simulink model "A_Justo_SCHFV_slx_IV"  (R2019a)
settings: Solver=VariableStepAuto  StartTime=0.0  StopTime=tfinal  MaxStep=maxstepsize  RelTol=1e-3  EnableMultiTasking=on
values from neighbouring files (symbols this model uses):
  aini = 0    [A_Justo_SCHFV_m_UFHDV_Design.m]
  B = [0; 0; 0; 0; 1/Tau_A]    [A_Justo_SCHFV_m_Control_Sensitivity.m]    (also in A_Justo_SCHFV_m_UFHDV_Design.m; TransferFunctionPROP.m)
  IDM_Amax = IDM_Amax(acc1+n1,acc1+n1)    [TransferFunctionPROP.m]
  IDM_Delta = IDM_Delta(acc1+n1)    [TransferFunctionPROP.m]
  IDM_H0 = IDM_H0(acc1+n1)    [TransferFunctionPROP.m]
  IDM_T = normrnd(IDM_t,IDM_ts)    [A_Justo_SCHFV_m_Control_Sensitivity.m]    (also in A_Justo_SCHFV_m_Track.m = IDM_Tind; A_Justo_SCHFV_m_UFHDV_Design.m; TransferFunctionPROP.m = IDM_T(acc1+n1,acc1+n1))
  IDM_V0 = IDM_V0(acc1+n1)    [TransferFunctionPROP.m]
  L = Lini    [A_Justo_SCHFV_m_Track.m]
  N = 11    [A_Justo_SCHFV_m_IV.m]    (also in A_Justo_SCHFV_m_Track.m)
  R = d/(2*pi)    (= 31.8309886184)    [A_Justo_SCHFV_m_IV.m]    (also in A_Justo_SCHFV_m_Track.m)
  Sidm = diag(isIDM)    [A_Justo_SCHFV_m_IV.m]    (also in A_Justo_SCHFV_m_Track.m)
  Smit = diag(isMIT)    [A_Justo_SCHFV_m_IV.m]    (also in A_Justo_SCHFV_m_Track.m)
  vini = 0    [A_Justo_SCHFV_m_UFHDV_Design.m]
undefined symbols (not defined in the file or in its folder): Bv, IDM_iSqab, iTau, MITSIM_a_Free_bra_high, MITSIM_a_Free_bra_low, MITSIM_a_Free_bra_mid, MITSIM_a_Free_bra_midhigh, MITSIM_a_Free_bra_midlow, MITSIM_a_Free_thr_high, MITSIM_a_Free_thr_low, MITSIM_a_Free_thr_mid, MITSIM_Alpha_bra, MITSIM_Alpha_thr, MITSIM_Beta_bra, MITSIM_Beta_thr, MITSIM_Gamma_bra, MITSIM_Gamma_thr, MITSIM_T_lower, MITSIM_T_upper, thini
settings Model: Creator=arnaudoria  LastModifiedBy=Sander
settings DataIOCC: LimitDataPoints=on  ReturnWorkspaceOutputs=off
settings OptimizationCC: LifeSpan=inf
settings DebuggingCC: AllowSymbolicDim=off  SFUnexpectedBacktrackingDiag=warning  SFNoUnconditionalDefaultTransitionDiag=warning  SFExecutionAtInitializationDiag=none  ArithmeticOperatorsInVariantConditions=warning
settings ModelReferenceCC: PropagateSignalLabelsOutOfModel=off
settings SFSimCC: SimUseLocalCustomCode=off
settings RTWCC: RTWUseLocalCustomCode=off
settings CodeAppCC: StateflowObjectComments=on
settings GRTTargetCC: TargetLangStandard=C89/C90 (ANSI)
settings ConfigComp: CovMetricSettings=dw  CovHtmlReporting=on  CovSaveCumulativeToWorkspaceVar=on  CovSaveSingleToWorkspaceVar=on  CovExternalEMLEnable=off

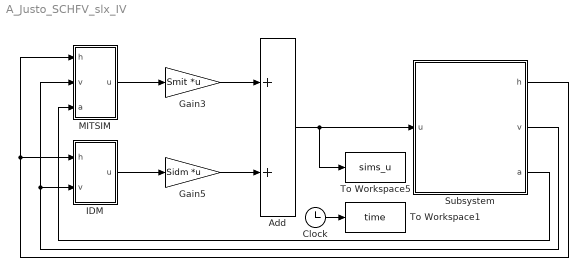
== system A_Justo_SCHFV_slx_IV ==
  Add : Sum
  Clock : Clock
  Gain3 : Gain  Gain=Smit  Multiplication=Matrix(K*u)
  Gain5 : Gain  Gain=Sidm  Multiplication=Matrix(K*u)
  IDM : Subsystem
  MITSIM : Subsystem
  Subsystem : Subsystem
  To Workspace1 : ToWorkspace  VariableName=time  SampleTime=-1
  To Workspace5 : ToWorkspace  VariableName=sims_u  SampleTime=-1
  wires:
  Clock/1 -> To Workspace1/1
  Subsystem/1(h) -> MITSIM/1(h), IDM/1(h)
  Subsystem/2(v) -> IDM/2(v), MITSIM/2(v)
  Subsystem/3(a) -> MITSIM/3(a)
  Add/1 -> Subsystem/1(u), To Workspace5/1
  Gain5/1 -> Add/2
  IDM/1(u) -> Gain5/1
  MITSIM/1(u) -> Gain3/1
  Gain3/1 -> Add/1

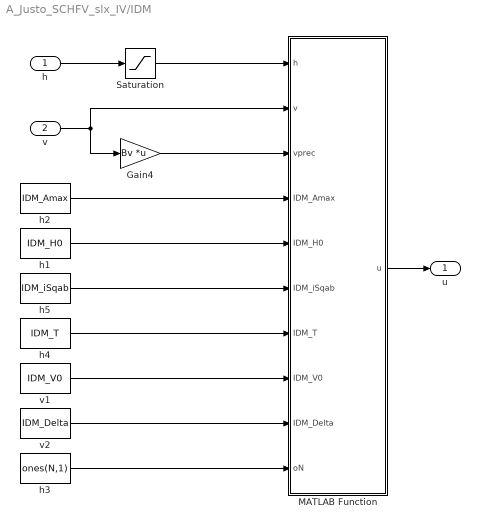
== system A_Justo_SCHFV_slx_IV/IDM ==
  h : Inport
  v : Inport  Port=2
  Gain4 : Gain  Gain=Bv  Multiplication=Matrix(K*u)
  MATLAB Function : MATLAB Function  TreatAsAtomicUnit=on
  Saturation : Saturate  UpperLimit=inf  LowerLimit=0.1
  h1 : Constant  Value=IDM_H0
  h2 : Constant  Value=IDM_Amax
  h3 : Constant  Value=ones(N,1)
  h4 : Constant  Value=IDM_T
  h5 : Constant  Value=IDM_iSqab
  v1 : Constant  Value=IDM_V0
  v2 : Constant  Value=IDM_Delta
  u : Outport
  wires:
  v/1 -> Gain4/1, MATLAB Function/2(v)
  v2/1 -> MATLAB Function/9(IDM_Delta)
  Gain4/1 -> MATLAB Function/3(vprec)
  h5/1 -> MATLAB Function/6(IDM_iSqab)
  MATLAB Function/1(u) -> u/1
  h4/1 -> MATLAB Function/7(IDM_T)
  h3/1 -> MATLAB Function/10(oN)
  Saturation/1 -> MATLAB Function/1(h)
  h/1 -> Saturation/1
  h1/1 -> MATLAB Function/5(IDM_H0)
  v1/1 -> MATLAB Function/8(IDM_V0)
  h2/1 -> MATLAB Function/4(IDM_Amax)

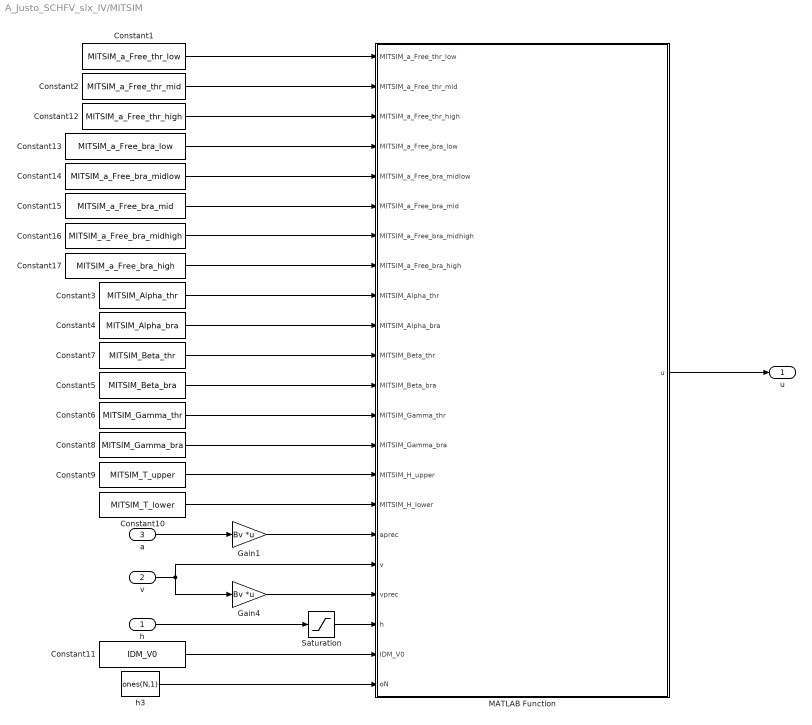
== system A_Justo_SCHFV_slx_IV/MITSIM ==
  h : Inport
  v : Inport  Port=2
  a : Inport  Port=3
  Constant1 : Constant  Value=MITSIM_a_Free_thr_low
  Constant10 : Constant  Value=MITSIM_T_lower
  Constant11 : Constant  Value=IDM_V0
  Constant12 : Constant  Value=MITSIM_a_Free_thr_high
  Constant13 : Constant  Value=MITSIM_a_Free_bra_low
  Constant14 : Constant  Value=MITSIM_a_Free_bra_midlow
  Constant15 : Constant  Value=MITSIM_a_Free_bra_mid
  Constant16 : Constant  Value=MITSIM_a_Free_bra_midhigh
  Constant17 : Constant  Value=MITSIM_a_Free_bra_high
  Constant2 : Constant  Value=MITSIM_a_Free_thr_mid
  Constant3 : Constant  Value=MITSIM_Alpha_thr
  Constant4 : Constant  Value=MITSIM_Alpha_bra
  Constant5 : Constant  Value=MITSIM_Beta_bra
  Constant6 : Constant  Value=MITSIM_Gamma_thr
  Constant7 : Constant  Value=MITSIM_Beta_thr
  Constant8 : Constant  Value=MITSIM_Gamma_bra
  Constant9 : Constant  Value=MITSIM_T_upper
  Gain1 : Gain  Gain=Bv  Multiplication=Matrix(K*u)
  Gain4 : Gain  Gain=Bv  Multiplication=Matrix(K*u)
  MATLAB Function : MATLAB Function  TreatAsAtomicUnit=on
  Saturation : Saturate  UpperLimit=inf  LowerLimit=0.1
  h3 : Constant  Value=ones(N,1)
  u : Outport
  wires:
  Saturation/1 -> MATLAB Function/20(h)
  h/1 -> Saturation/1
  MATLAB Function/1(u) -> u/1
  Gain4/1 -> MATLAB Function/19(vprec)
  v/1 -> Gain4/1, MATLAB Function/18(v)
  Constant1/1 -> MATLAB Function/1(MITSIM_a_Free_thr_low)
  Constant2/1 -> MATLAB Function/2(MITSIM_a_Free_thr_mid)
  Constant3/1 -> MATLAB Function/9(MITSIM_Alpha_thr)
  h3/1 -> MATLAB Function/22(oN)
  a/1 -> Gain1/1
  Gain1/1 -> MATLAB Function/17(aprec)
  Constant4/1 -> MATLAB Function/10(MITSIM_Alpha_bra)
  Constant7/1 -> MATLAB Function/11(MITSIM_Beta_thr)
  Constant5/1 -> MATLAB Function/12(MITSIM_Beta_bra)
  Constant6/1 -> MATLAB Function/13(MITSIM_Gamma_thr)
  Constant8/1 -> MATLAB Function/14(MITSIM_Gamma_bra)
  Constant9/1 -> MATLAB Function/15(MITSIM_H_upper)
  Constant10/1 -> MATLAB Function/16(MITSIM_H_lower)
  Constant11/1 -> MATLAB Function/21(IDM_V0)
  Constant12/1 -> MATLAB Function/3(MITSIM_a_Free_thr_high)
  Constant13/1 -> MATLAB Function/4(MITSIM_a_Free_bra_low)
  Constant14/1 -> MATLAB Function/5(MITSIM_a_Free_bra_midlow)
  Constant15/1 -> MATLAB Function/6(MITSIM_a_Free_bra_mid)
  Constant16/1 -> MATLAB Function/7(MITSIM_a_Free_bra_midhigh)
  Constant17/1 -> MATLAB Function/8(MITSIM_a_Free_bra_high)

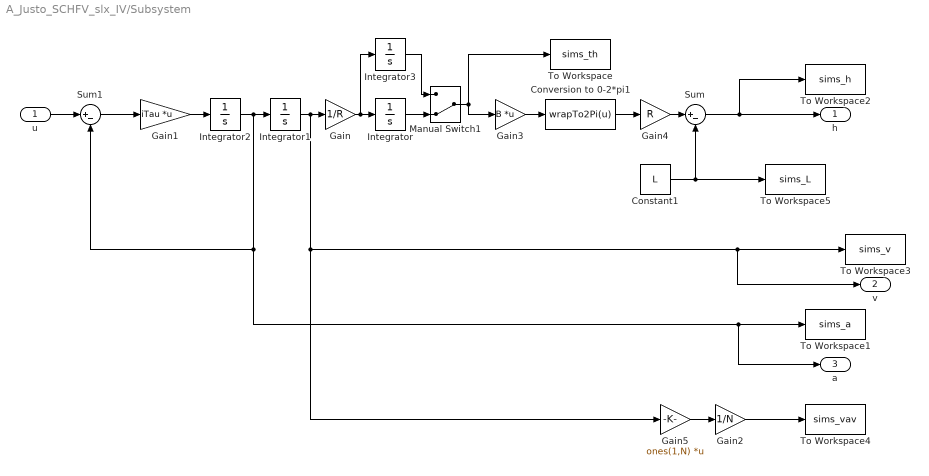
== system A_Justo_SCHFV_slx_IV/Subsystem ==
  u : Inport
  Constant1 : Constant  Value=L
  Conversion to 0-2*pi1 : MATLABFcn  MATLABFcn=wrapTo2Pi(u)
  Gain : Gain  Gain=1/R
  Gain1 : Gain  Gain=iTau  Multiplication=Matrix(K*u)
  Gain2 : Gain  Gain=1/N
  Gain3 : Gain  Gain=B  Multiplication=Matrix(K*u)
  Gain4 : Gain  Gain=R
  Gain5 : Gain  Gain=ones(1,N)  Multiplication=Matrix(K*u)
  Integrator : Integrator  InitialCondition=thini  WrapState=on  WrappedStateUpperValue=2*pi  WrappedStateLowerValue=0
  Integrator1 : Integrator  InitialCondition=vini  LimitOutput=on  LowerSaturationLimit=0  WrappedStateUpperValue=2*pi  WrappedStateLowerValue=0
  Integrator2 : Integrator  InitialCondition=aini  WrappedStateUpperValue=2*pi  WrappedStateLowerValue=0
  Integrator3 : Integrator  InitialCondition=thini  WrappedStateUpperValue=2*pi  WrappedStateLowerValue=0
  Manual Switch1 : ManualSwitch  CurrentSetting=0
  Sum : Sum  Inputs=|+-
  Sum1 : Sum  Inputs=|+-
  To Workspace : ToWorkspace  VariableName=sims_th  SampleTime=-1
  To Workspace1 : ToWorkspace  VariableName=sims_a  SampleTime=-1
  To Workspace2 : ToWorkspace  VariableName=sims_h  SampleTime=-1
  To Workspace3 : ToWorkspace  VariableName=sims_v  SampleTime=-1
  To Workspace4 : ToWorkspace  VariableName=sims_vav  SampleTime=-1
  To Workspace5 : ToWorkspace  VariableName=sims_L  SampleTime=-1
  h : Outport
  v : Outport  Port=2
  a : Outport  Port=3
  wires:
  Gain/1 -> Integrator3/1, Integrator/1
  Gain3/1 -> Conversion to 0-2*pi1/1
  Gain4/1 -> Sum/1
  Sum/1 -> To Workspace2/1, h/1
  u/1 -> Sum1/1
  Integrator1/1 -> Gain5/1, v/1, To Workspace3/1, Gain/1
  Integrator2/1 -> To Workspace1/1, a/1, Sum1/2, Integrator1/1
  Gain1/1 -> Integrator2/1
  Sum1/1 -> Gain1/1
  Integrator3/1 -> Manual Switch1/1
  Integrator/1 -> Manual Switch1/2
  Manual Switch1/1 -> To Workspace/1, Gain3/1
  Conversion to 0-2*pi1/1 -> Gain4/1
  Gain5/1 -> Gain2/1
  Gain2/1 -> To Workspace4/1
  Constant1/1 -> To Workspace5/1, Sum/2

== matlab function A_Justo_SCHFV_slx_IV/IDM/MATLAB Function ==
  data: h input; v input; vprec input; IDM_Amax input; IDM_H0 input; IDM_iSqab input; IDM_T input; IDM_V0 input; IDM_Delta input; u output; oN input
function u = fcn(h,v,vprec,IDM_Amax,IDM_H0,IDM_iSqab,IDM_T,IDM_V0,IDM_Delta,oN)

% IDM
hr = IDM_H0+max(oN*0,IDM_T*v+v.*(v-vprec).*IDM_iSqab);
% Condition for avoiding numerical errors
v = v.*(v>0);
% Control
u = IDM_Amax*(oN-(v./IDM_V0).^IDM_Delta-(hr./h).^2);

== matlab function A_Justo_SCHFV_slx_IV/MITSIM/MATLAB Function ==
  data: MITSIM_a_Free_thr_low input; MITSIM_a_Free_thr_mid input; MITSIM_a_Free_thr_high input; MITSIM_a_Free_bra_low input; MITSIM_a_Free_bra_midlow input; MITSIM_a_Free_bra_mid input; MITSIM_a_Free_bra_midhigh input; MITSIM_a_Free_bra_high input; MITSIM_Alpha_thr input; MITSIM_Alpha_bra input; MITSIM_Beta_thr input; MITSIM_Beta_bra input; MITSIM_Gamma_thr input; MITSIM_Gamma_bra input; MITSIM_H_upper input; MITSIM_H_lower input; aprec input; v input; vprec input; h input; IDM_V0 input; u output; oN input
function u = fcn(MITSIM_a_Free_thr_low, MITSIM_a_Free_thr_mid, ...
    MITSIM_a_Free_thr_high, MITSIM_a_Free_bra_low, ...
    MITSIM_a_Free_bra_midlow, MITSIM_a_Free_bra_mid, ...
    MITSIM_a_Free_bra_midhigh, MITSIM_a_Free_bra_high, MITSIM_Alpha_thr...
    , MITSIM_Alpha_bra, MITSIM_Beta_thr, MITSIM_Beta_bra, ...
MITSIM_Gamma_thr, MITSIM_Gamma_bra, MITSIM_H_upper, MITSIM_H_lower, ...
aprec, v, vprec, h, IDM_V0, oN)

if isempty(find(h<=0, 1))==0  % Display a message to show when some h is not positive
    error('Vehicles have crashed. Simulation has been stopped.')
end

hd_tm = h./v;

% Obtain the indexes that correspond to each regime
ind_free_thr_low = hd_tm>MITSIM_H_upper & v<IDM_V0 & v>12.192;
ind_free_thr_mid = hd_tm>MITSIM_H_upper & v<IDM_V0 & v<=12.192 & v>=6.096;
ind_free_thr_high = hd_tm>MITSIM_H_upper & v<IDM_V0 & v<6.096;
ind_free_zro = hd_tm>MITSIM_H_upper & v==IDM_V0;
ind_free_bra_low = hd_tm>MITSIM_H_upper & v>IDM_V0 & v>24.4;
ind_free_bra_midlow = hd_tm>MITSIM_H_upper & v>IDM_V0 & v>=18.3 & v<=24.4;
ind_free_bra_mid = hd_tm>MITSIM_H_upper & v>IDM_V0 & v>=12.2 & v<18.3;
ind_free_bra_midhigh = hd_tm>MITSIM_H_upper & v>IDM_V0 & v>=6.1 & v<12.2;
ind_free_bra_high = hd_tm>MITSIM_H_upper & v>IDM_V0 & v<6.1;

ind_fllw_thr = hd_tm>=MITSIM_H_lower & hd_tm<=MITSIM_H_upper & v<=vprec;
ind_fllw_bra = hd_tm>=MITSIM_H_lower & hd_tm<=MITSIM_H_upper & v>vprec;

ind_emer_thr_low = hd_tm<MITSIM_H_lower & v<=vprec & v>24.4;
ind_emer_thr_midlow = hd_tm<MITSIM_H_lower & v<=vprec & v>=18.3 & v<=24.4;
ind_emer_thr_mid = hd_tm<MITSIM_H_lower & v<=vprec & v>=12.2 & v<18.3;
ind_emer_thr_midhigh = hd_tm<MITSIM_H_lower & v<=vprec & v>=6.1 & v<12.2;
ind_emer_thr_high = hd_tm<MITSIM_H_lower & v<=vprec & v<6.1;
ind_emer_bra_low = hd_tm<MITSIM_H_lower & v>vprec & v>24.4;
ind_emer_bra_midlow = hd_tm<MITSIM_H_lower & v>vprec & v>=18.3 & v<=24.4;
ind_emer_bra_mid = hd_tm<MITSIM_H_lower & v>vprec & v>=12.2 & v<18.3;
ind_emer_bra_midhigh = hd_tm<MITSIM_H_lower & v>vprec & v>=6.1 & v<12.2;
ind_emer_bra_high = hd_tm<MITSIM_H_lower & v>vprec & v<6.1;

% Control
u=oN*0;
% Condition for avoiding numerical errors
v = v.*(v>0);

% MITSIM - Free driving
u(ind_free_thr_low) = MITSIM_a_Free_thr_low(ind_free_thr_low,...
    ind_free_thr_low)*oN(ind_free_thr_low);
u(ind_free_thr_mid) = MITSIM_a_Free_thr_mid(ind_free_thr_mid,...
    ind_free_thr_mid)*oN(ind_free_thr_mid);
u(ind_free_thr_high) = MITSIM_a_Free_thr_high(ind_free_thr_high,...
    ind_free_thr_high)*oN(ind_free_thr_high);
u(ind_free_zro) = 0*oN(ind_free_zro);
u(ind_free_bra_low) = MITSIM_a_Free_bra_low(ind_free_bra_low,...
    ind_free_bra_low)*oN(ind_free_bra_low);
u(ind_free_bra_midlow) = MITSIM_a_Free_bra_midlow(ind_free_bra_midlow,...
    ind_free_bra_midlow)*oN(ind_free_bra_midlow);
u(ind_free_bra_mid) = MITSIM_a_Free_bra_mid(ind_free_bra_mid,...
    ind_free_bra_mid)*oN(ind_free_bra_mid);
u(ind_free_bra_midhigh) = MITSIM_a_Free_bra_midhigh(ind_free_bra_midhigh,...
    ind_free_bra_midhigh)*oN(ind_free_bra_midhigh);
u(ind_free_bra_high) = MITSIM_a_Free_bra_high(ind_free_bra_high,...
    ind_free_bra_high)*oN(ind_free_bra_high);

% MITSIM - Following regime
u(ind_fllw_thr) = MITSIM_Alpha_thr(ind_fllw_thr,ind_fllw_thr)*...
    (v(ind_fllw_thr).^MITSIM_Beta_thr(ind_fllw_thr).*...
    (vprec(ind_fllw_thr)-v(ind_fllw_thr))./h(ind_fllw_thr).^...
    MITSIM_Gamma_thr(ind_fllw_thr));
u(ind_fllw_bra) = MITSIM_Alpha_bra(ind_fllw_bra,ind_fllw_bra)*...
    (v(ind_fllw_bra).^MITSIM_Beta_bra(ind_fllw_bra).*...
    (vprec(ind_fllw_bra)-v(ind_fllw_bra))./h(ind_fllw_bra).^...
    MITSIM_Gamma_bra(ind_fllw_bra));

% MITSIM - Emergency brake
u(ind_emer_thr_low) = min(MITSIM_a_Free_bra_low(ind_emer_thr_low,...
    ind_emer_thr_low)*oN(ind_emer_thr_low),aprec(ind_emer_thr_low)...
    +0.25*MITSIM_a_Free_bra_low(ind_emer_thr_low,ind_emer_thr_low)...
    *oN(ind_emer_thr_low));
u(ind_emer_thr_midlow) = min(MITSIM_a_Free_bra_midlow(ind_emer_thr_midlow,...
    ind_emer_thr_midlow)*oN(ind_emer_thr_midlow),aprec(ind_emer_thr_midlow)...
    +0.25*MITSIM_a_Free_bra_midlow(ind_emer_thr_midlow,ind_emer_thr_midlow)...
    *oN(ind_emer_thr_midlow));
u(ind_emer_thr_mid) = min(MITSIM_a_Free_bra_mid(ind_emer_thr_mid,...
    ind_emer_thr_mid)*oN(ind_emer_thr_mid),aprec(ind_emer_thr_mid)...
    +0.25*MITSIM_a_Free_bra_mid(ind_emer_thr_mid,ind_emer_thr_mid)...
    *oN(ind_emer_thr_mid));
u(ind_emer_thr_midhigh) = min(MITSIM_a_Free_bra_midhigh(ind_emer_thr_midhigh,...
    ind_emer_thr_midhigh)*oN(ind_emer_thr_midhigh),aprec(ind_emer_thr_midhigh)...
    +0.25*MITSIM_a_Free_bra_midhigh(ind_emer_thr_midhigh,ind_emer_thr_midhigh)...
    *oN(ind_emer_thr_midhigh));
u(ind_emer_thr_high) = min(MITSIM_a_Free_bra_high(ind_emer_thr_high,...
    ind_emer_thr_high)*oN(ind_emer_thr_high),aprec(ind_emer_thr_high)...
    +0.25*MITSIM_a_Free_bra_high(ind_emer_thr_high,ind_emer_thr_high)...
    *oN(ind_emer_thr_high));
u(ind_emer_bra_low) = min(MITSIM_a_Free_bra_low(ind_emer_bra_low,...
    ind_emer_bra_low)*oN(ind_emer_bra_low),aprec(ind_emer_bra_low)...
    -0.5*(v(ind_emer_bra_low)-vprec(ind_emer_bra_low))...
    .^2./h(ind_emer_bra_low));
u(ind_emer_bra_midlow) = min(MITSIM_a_Free_bra_midlow(ind_emer_bra_midlow,...
    ind_emer_bra_midlow)*oN(ind_emer_bra_midlow),aprec(ind_emer_bra_midlow)...
    -0.5*(v(ind_emer_bra_midlow)-vprec(ind_emer_bra_midlow))...
    .^2./h(ind_emer_bra_midlow));
u(ind_emer_bra_mid) = min(MITSIM_a_Free_bra_mid(ind_emer_bra_mid,...
    ind_emer_bra_mid)*oN(ind_emer_bra_mid),aprec(ind_emer_bra_mid)...
    -0.5*(v(ind_emer_bra_mid)-vprec(ind_emer_bra_mid))...
    .^2./h(ind_emer_bra_mid));
u(ind_emer_bra_midhigh) = min(MITSIM_a_Free_bra_midhigh(ind_emer_bra_midhigh,...
    ind_emer_bra_midhigh)*oN(ind_emer_bra_midhigh),aprec(ind_emer_bra_midhigh)...
    -0.5*(v(ind_emer_bra_midhigh)-vprec(ind_emer_bra_midhigh))...
    .^2./h(ind_emer_bra_midhigh));
u(ind_emer_bra_high) = min(MITSIM_a_Free_bra_high(ind_emer_bra_high,...
    ind_emer_bra_high)*oN(ind_emer_bra_high),aprec(ind_emer_bra_high)...
    -0.5*(v(ind_emer_bra_high)-vprec(ind_emer_bra_high))...
    .^2./h(ind_emer_bra_high));
end
